simulink model "Vehicle_suspension"  (R2020b)
settings: Solver=VariableStepAuto  StartTime=0.0  StopTime=100  RelTol=1e-3
values from neighbouring files (symbols this model uses):
  b = 350.0    [data_dict.sldd]
  k1 = 80000.0    [data_dict.sldd]
  k2 = 500000.0    [data_dict.sldd]
  M1 = 2500.0    [data_dict.sldd]
  M2 = 320.0    [data_dict.sldd]
settings Model: DataDictionary=data_dict.sldd  Creator=Shree  LastModifiedBy=Shree
settings DataIOCC: ExternalInput=[t, stin]  LoadExternalInput=on

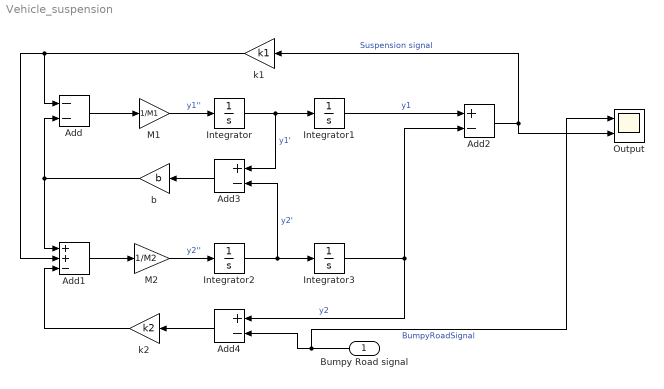
== system Vehicle_suspension ==
  Bumpy Road signal : Inport
  Add : Sum  Inputs=--
  Add1 : Sum  Inputs=++-
  Add2 : Sum  Inputs=+-
  Add3 : Sum  Inputs=+-
  Add4 : Sum  Inputs=+-
  Integrator{,1..3} (4 alike) : Integrator
  M1 : Gain  Gain=1/M1
  M2 : Gain  Gain=1/M2
  Output : Scope  NumInputPorts=2
  b : Gain  Gain=b
  k1 : Gain  Gain=k1
  k2 : Gain  Gain=k2
  wires:
  Add/1 -> M1/1
  M1/1 -> Integrator/1  "y1''"
  Integrator2/1 -> Add3/2, Integrator3/1  "y2'"
  Add1/1 -> M2/1
  M2/1 -> Integrator2/1  "y2''"
  Integrator1/1 -> Add2/1  "y1"
  Integrator3/1 -> Add4/1, Add2/2  "y2"
  Add2/1 -> Output/2, k1/1  "Suspension signal"
  k1/1 -> Add1/2, Add/1
  Integrator/1 -> Add3/1, Integrator1/1  "y1'"
  Add3/1 -> b/1
  b/1 -> Add1/1, Add/2
  k2/1 -> Add1/3
  Add4/1 -> k2/1
  Bumpy Road signal/1 -> Output/1, Add4/2  "BumpyRoadSignal"
